simulink model "SAD_library"  (R2023b)
settings: Solver=VariableStepAuto  StartTime=0.0  StopTime=10.0  RelTol=1e-3
values from neighbouring files (symbols this model uses):
  A = 1e-2.*[6, 6, 6, 6, 4, 4, 12, 12, 12, 12]'    [SAD_project_code.m]
  e = 0.001    [SAD_project_code.m]
  FS = 800e-9    (= 8e-07)    [SAD_project_code.m]
  i = deg2rad(60)    [SAD_project_code.m]
  inc_tot = sqrt(inc_lin^2 + inc_acc^2)    [SAD_project_code.m]
  p = a*(1-e^2)    [SAD_project_code.m]
  R_E = astroConstants(23)    [SAD_project_code.m]
  ts_sensor = t_step    (= 0.01)    [SAD_project_code.m]
  w_E = deg2rad(15.04)/60/60    [SAD_project_code.m]
undefined symbols (not defined in the file or in its folder): A_1, A_10, A_2, A_3, A_4, A_5, A_6, A_7, A_8, A_9, gain_thdot, N_1, N_10, N_2, N_3, N_4, N_5, N_6, N_7, N_8, N_9, r_1, r_10, r_2, r_3, r_4, r_5, r_6, r_7, r_8, r_9, rho_d1, rho_d10, rho_d2, rho_d3, rho_d4, rho_d5, rho_d6, rho_d7, rho_d8, rho_d9, rho_s1, rho_s10, rho_s2, rho_s3, rho_s4, rho_s5, rho_s6, rho_s7, rho_s8, rho_s9
libraries: matrix_library x11
settings Model: Creator=samue  LastModifiedBy=rkomiii_masca

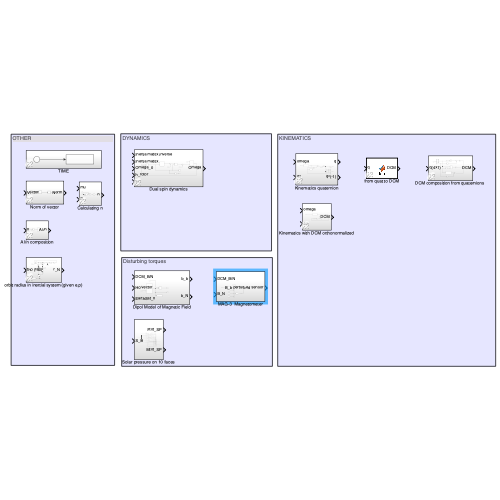
[thumbnail: Simulink's stored preview of the top-level diagram]
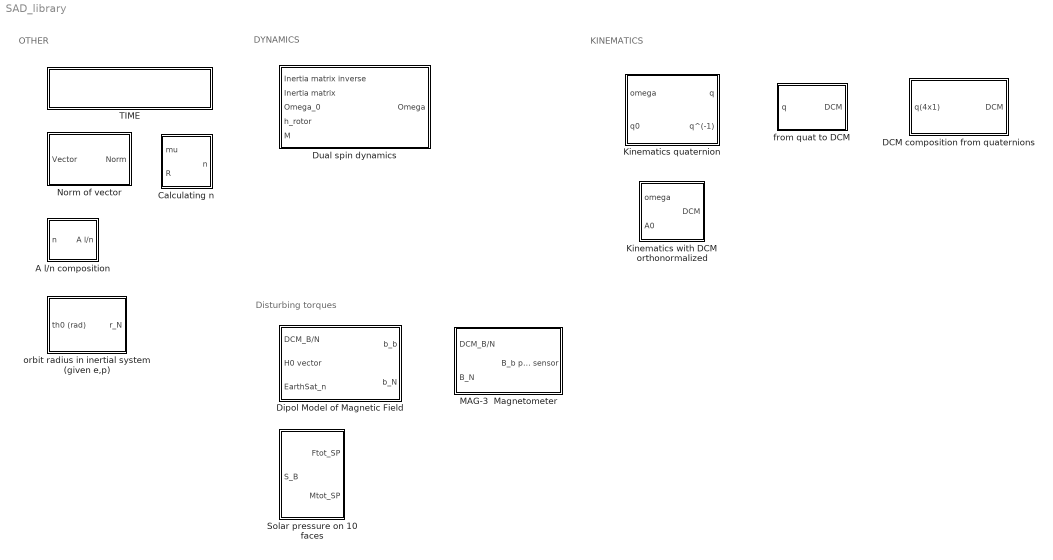
== system SAD_library ==
  note: KINEMATICS
  note: Disturbing torques
  note: OTHER
  note: DYNAMICS
  A l/n composition : Subsystem  AncestorBlock=LibrarySAD5/A l//n composition
  Calculating n : Subsystem  AncestorBlock=LibrarySAD5/Calculating n
  "DCM composition from quaternions " : Subsystem  AncestorBlock=LibrarySAD5/DCM composition from quaternions
  Dipol Model of Magnetic Field : Subsystem
  Dual spin dynamics : Subsystem  AncestorBlock=LibrarySAD5/Dual spin dynamics
  Kinematics quaternion : Subsystem  AncestorBlock=LibrarySAD5/Kinematics quaternion
  Kinematics with DCM orthonormalized : Subsystem  AncestorBlock=LibrarySAD5/Kinematics with DCM orthonormalized
  MAG-3  Magnetometer : Subsystem
  Norm of vector : Subsystem  AncestorBlock=LibrarySAD5/Normalize Vector1
  Solar pressure on 10 faces : Subsystem
  TIME : Subsystem  AncestorBlock=LibrarySAD5/TIME
  from quat to DCM : MATLAB Function  AncestorBlock=LibrarySAD5/from quat to DCM  TreatAsAtomicUnit=on
  orbit radius in inertial system (given e,p) : Subsystem  AncestorBlock=LibrarySAD5/orbit radius in inertial system (given e,p)

== system SAD_library/A l//n composition ==
  n : Inport
  Clock : Clock
  Product : Product
  Rotation matrix 3 : Subsystem
  A l/n : Outport
  wires:
  Rotation matrix 3/1(Out1) -> A l/n/1
  Product/1 -> Rotation matrix 3/1(In1)
  n/1 -> Product/1
  Clock/1 -> Product/2

== system SAD_library/Calculating n ==
  mu : Inport
  R : Inport  Port=2
  Divide : Product  Inputs=*/
  Product : Product  Inputs=3
  Sqrt : Sqrt
  n : Outport
  wires:
  Product/1 -> Divide/2
  Sqrt/1 -> n/1
  Divide/1 -> Sqrt/1
  mu/1 -> Divide/1
  R/1 -> Product/3, Product/2, Product/1

== system SAD_library/DCM composition from quaternions  ==
  q(4x1) : Inport
  Cross product matrix composition : Subsystem
  Demux : Demux
  Dot Product : DotProduct  OutDataTypeStr=Inherit: Inherit via internal rule
  Gain : Gain  Gain=[1 0 0; 0 1 0; 0 0 1]
  Gain1 : Gain  Gain=2
  Gain2 : Gain  Gain=-2
  Mux : Mux  Inputs=3
  Product : Product  Multiplication=Matrix(*)
  Product1 : Product
  Square : Math  Operator=square
  Sum : Sum  Inputs=|-+
  Sum1 : Sum  Inputs=+++
  Transpose : Math  Operator=transpose
  DCM : Outport
  wires:
  Gain/1 -> Sum1/1
  Demux/1 -> Mux/1
  q(4x1)/1 -> Demux/1
  Demux/2 -> Mux/2
  Mux/1 -> Dot Product/2, Dot Product/1, Product/1, Cross product matrix composition/1(q_vect), Transpose/1  "q_vect"
  Demux/4 -> Gain2/1, Square/1  "q4"
  Demux/3 -> Mux/3
  Dot Product/1 -> Sum/1
  Sum/1 -> Gain/1
  Square/1 -> Sum/2
  Transpose/1 -> Product/2
  Product/1 -> Gain1/1
  Gain2/1 -> Product1/2
  Cross product matrix composition/1(q_vect cross) -> Product1/1  "omega_mat"
  Product1/1 -> Sum1/3
  Gain1/1 -> Sum1/2
  Sum1/1 -> DCM/1

== system SAD_library/Dipol Model of Magnetic Field ==
  note: CODE TO ADD
      | % Definition of Magnetic Field (Dipole model)
      |  j_b = [0.01 0.05 0.01]';
      | H0 = 1e-9.*[-29404.8 -1450.9 4652.5]';
  DCM_B/N : Inport
  H0 vector : Inport  Port=2
  EarthSat_n : Inport  Port=3
  Calculation of b_n : Subsystem
  Matrix Multiply : Product  Multiplication=Matrix(*)
  To Workspace : ToWorkspace  VariableName=bn  SampleTime=-1
  b_b : Outport
  b_N : Outport  Port=2
  wires:
  Matrix Multiply/1 -> b_b/1
  DCM_B/N/1 -> Matrix Multiply/1
  H0 vector/1 -> Calculation of b_n/1(H0 vector)
  EarthSat_n/1 -> Calculation of b_n/2(EarthSat_n)
  Calculation of b_n/1(b_N) -> To Workspace/1, b_N/1, Matrix Multiply/2

== system SAD_library/Dual spin dynamics ==
  Inertia matrix inverse : Inport
  Inertia matrix : Inport  Port=2
  Omega_0 : Inport  Port=3
  h_rotor : Inport  Port=4
  M : Inport  Port=5
  Cross Product1 : matrix_library/Cross Product
  Integrator1 : Integrator  InitialConditionSource=external
  Product2 : Product  Multiplication=Matrix(*)
  Product3 : Product  Multiplication=Matrix(*)
  Scope2 : Scope
  Sum : Sum  Inputs=|++
  Sum1 : Sum  Inputs=|++
  Transpose : Math  Operator=transpose
  Omega : Outport
  wires:
  M/1 -> Sum1/2
  Sum1/1 -> Product3/2
  Omega_0/1 -> Integrator1/2
  Product2/1 -> Sum/1  "h"
  Inertia matrix/1 -> Product2/1
  Product3/1 -> Integrator1/1  "d_om/dt"
  h_rotor/1 -> Sum/2
  Integrator1/1 -> Product2/2, Cross Product1/2, Scope2/1, Transpose/1  "omega"
  Cross Product1/1 -> Sum1/1
  Inertia matrix inverse/1 -> Product3/1
  Sum/1 -> Cross Product1/1
  Transpose/1 -> Omega/1

== system SAD_library/Kinematics quaternion ==
  omega : Inport
  q0 : Inport  Port=2
  Demux : Demux
  Divide : Product  Inputs=*/
  Gain1 : Gain  Gain=-1
  Gain2 : Gain  Gain=-1
  Gain3 : Gain  Gain=1/2
  Gain5 : Gain  Gain=-1
  Integrator : Integrator  InitialConditionSource=external
  Matrix Multiply : Product  Multiplication=Matrix(*)
  Matrix OMEGA : Subsystem
  Mux : Mux
  Norm of Vector : Subsystem
  Scope : Scope
  q : Outport
  q^(-1) : Outport  Port=2
  wires:
  Gain3/1 -> Matrix Multiply/1  "1/2*Omega"
  Matrix Multiply/1 -> Integrator/1  "dq/dt"
  omega/1 -> Matrix OMEGA/1(omega)
  Integrator/1 -> Scope/1, q/1, Norm of Vector/1(Vector), Divide/1, Demux/1  "q"
  Matrix OMEGA/1(Matrix Omega) -> Gain3/1  "Omega"
  q0/1 -> Integrator/2
  Demux/2 -> Gain1/1
  Demux/3 -> Gain2/1
  Gain1/1 -> Mux/2
  Gain2/1 -> Mux/3
  Demux/4 -> Mux/4
  Mux/1 -> q^(-1)/1
  Norm of Vector/1(Norm) -> Divide/2  "q_norm"
  Divide/1 -> Matrix Multiply/2  "normalized q"
  Demux/1 -> Gain5/1
  Gain5/1 -> Mux/1

== system SAD_library/Kinematics with DCM orthonormalized ==
  omega : Inport
  A0 : Inport  Port=2
  Cross product matrix composition : Subsystem
  Integrator3 : Integrator  InitialConditionSource=external
  Orthonormalization of DCM : Subsystem
  Product1 : Product  Multiplication=Matrix(*)
  DCM : Outport
  wires:
  Integrator3/1 -> Orthonormalization of DCM/1(DCM), DCM/1  "DCM"
  Cross product matrix composition/1(omega cross) -> Product1/1  "omega cross"
  omega/1 -> Cross product matrix composition/1(omega)
  Orthonormalization of DCM/1(orthDCM) -> Product1/2
  Product1/1 -> Integrator3/1
  A0/1 -> Integrator3/2

== system SAD_library/MAG-3  Magnetometer ==
  note: CODE TO ADD TO MAKE SENSOR WORK
      | % Time definition
      | t0 = 0;
      | tf = T; %Period of orbit
      | t_step = 0.01; %fixed step of simulation
      | ts_sensor = t_step; % Sample of sensor (can change but must to be a multiple of t_step)
      |
      | % MAG-3 sensor data and error
      | FS = 500e-9; %Full scale value
      | inc_lin = 0.15/100; % Accuracy error
      | inc_acc = 0.75/100; % Linear error
      | inc_tot = sqrt(inc_lin^2 + inc_acc^2); %Total error
  DCM_B/N : Inport
  B_N : Inport  Port=2
  Error gain of sensor MAG-3 : Gain  Gain=inc_tot*FS
  Rotation in body frame : Product  Multiplication=Matrix(*)
  Sample of sensor : ZeroOrderHold  SampleTime=ts_sensor
  Saturation to FS : Saturate  UpperLimit=FS  LowerLimit=-FS
  Sum : Sum  Inputs=|++
  Vector Concatenate : Concatenate  NumInputs=3
  White Noise : RandomNumber  DisableCoverage=on  Seed=1  SampleTime=ts_sensor
  White Noise1 : RandomNumber  DisableCoverage=on  Seed=2  SampleTime=ts_sensor
  White Noise2 : RandomNumber  DisableCoverage=on  Seed=3  SampleTime=ts_sensor
  B_b perturbed sensor : Outport
  wires:
  Vector Concatenate/1 -> Error gain of sensor MAG-3/1
  White Noise/1 -> Vector Concatenate/1
  Error gain of sensor MAG-3/1 -> Sum/2
  White Noise2/1 -> Vector Concatenate/3
  White Noise1/1 -> Vector Concatenate/2
  Sum/1 -> Saturation to FS/1
  B_N/1 -> Sample of sensor/1
  DCM_B/N/1 -> Rotation in body frame/1
  Saturation to FS/1 -> B_b perturbed sensor/1
  Sample of sensor/1 -> Rotation in body frame/2
  Rotation in body frame/1 -> Sum/1

== system SAD_library/Norm of vector ==
  Vector : Inport
  Dot Product : DotProduct  OutDataTypeStr=Inherit: Inherit via internal rule
  Sqrt : Sqrt
  Norm : Outport
  wires:
  Sqrt/1 -> Norm/1
  Vector/1 -> Dot Product/1, Dot Product/2
  Dot Product/1 -> Sqrt/1

== system SAD_library/Solar pressure on 10 faces ==
  S_B : Inport
  Sum of forces : Sum  Inputs=++++++++++
  Sum of moments : Sum  Inputs=++++++++++
  solar pressure force and torque 1 : Subsystem
  solar pressure force and torque 10 : Subsystem
  solar pressure force and torque 2 : Subsystem
  solar pressure force and torque 3 : Subsystem
  solar pressure force and torque 4 : Subsystem
  solar pressure force and torque 5 : Subsystem
  solar pressure force and torque 6 : Subsystem
  solar pressure force and torque 7 : Subsystem
  solar pressure force and torque 8 : Subsystem
  solar pressure force and torque 9 : Subsystem
  Ftot_SP : Outport
  Mtot_SP : Outport  Port=2
  wires:
  solar pressure force and torque 1/1(F_1) -> Sum of forces/5
  solar pressure force and torque 2/1(F_2) -> Sum of forces/6
  solar pressure force and torque 3/1(F_3) -> Sum of forces/7
  solar pressure force and torque 4/1(F_4) -> Sum of forces/8
  solar pressure force and torque 5/1(F_5) -> Sum of forces/9
  solar pressure force and torque 6/1(F_6) -> Sum of forces/10
  solar pressure force and torque 7/1(F_7) -> Sum of forces/1
  solar pressure force and torque 8/1(F_8) -> Sum of forces/2
  solar pressure force and torque 9/1(F_9) -> Sum of forces/3
  solar pressure force and torque 10/1(F_10) -> Sum of forces/4
  solar pressure force and torque 1/2(M_1) -> Sum of moments/5
  solar pressure force and torque 2/2(M_2) -> Sum of moments/6
  solar pressure force and torque 3/2(M_3) -> Sum of moments/7
  solar pressure force and torque 4/2(M_4) -> Sum of moments/8
  solar pressure force and torque 5/2(M_5) -> Sum of moments/9
  solar pressure force and torque 6/2(M_6) -> Sum of moments/10
  solar pressure force and torque 7/2(M_7) -> Sum of moments/1
  solar pressure force and torque 8/2(M_8) -> Sum of moments/2
  solar pressure force and torque 9/2(M_9) -> Sum of moments/3
  solar pressure force and torque 10/2(M_10) -> Sum of moments/4
  Sum of forces/1 -> Ftot_SP/1  "Ftot_SP"
  Sum of moments/1 -> Mtot_SP/1  "Mtot_SP"
  S_B/1 -> solar pressure force and torque 10/1(s_B), solar pressure force and torque 9/1(s_B), solar pressure force and torque 6/1(s_B), solar pressure force and torque 5/1(s_B), solar pressure force and torque 4/1(s_B), solar pressure force and torque 7/1(s_B), solar pressure force and torque 8/1(s_B), solar pressure force and torque 1/1(s_B), solar pressure force and torque 2/1(s_B), solar pressure force and torque 3/1(s_B)

== system SAD_library/TIME ==
  Clock : Clock
  To Workspace1 : ToWorkspace  VariableName=t  SampleTime=-1
  wires:
  Clock/1 -> To Workspace1/1

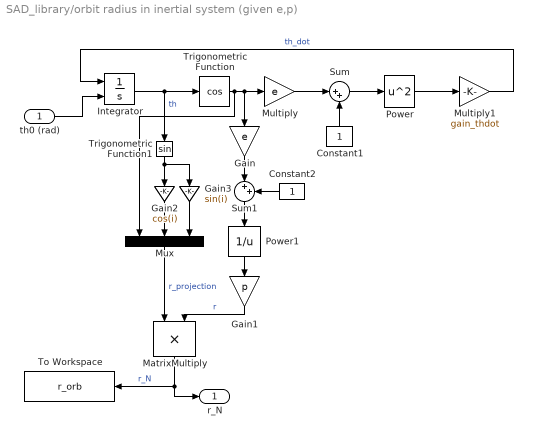
== system SAD_library/orbit radius in inertial system (given e,p) ==
  th0 (rad) : Inport
  Constant1 : Constant
  Constant2 : Constant
  Gain : Gain  Gain=e
  Gain1 : Gain  Gain=p
  Gain2 : Gain  Gain=cos(i)
  Gain3 : Gain  Gain=sin(i)
  Integrator : Integrator  InitialConditionSource=external
  MatrixMultiply : Product
  Multiply : Gain  Gain=e
  Multiply1 : Gain  Gain=gain_thdot
  Mux : Mux  Inputs=3
  Power : Math  Operator=square
  Power1 : Math  Operator=reciprocal
  Sum : Sum  Inputs=|++
  Sum1 : Sum  Inputs=|++
  To Workspace : ToWorkspace  VariableName=r_orb  SampleTime=-1
  Trigonometric Function : Trigonometry  Operator=cos
  Trigonometric Function1 : Trigonometry
  r_N : Outport
  wires:
  Mux/1 -> MatrixMultiply/1  "r_projection"
  Power1/1 -> Gain1/1
  Gain1/1 -> MatrixMultiply/2  "r"
  Gain2/1 -> Mux/2
  Sum1/1 -> Power1/1
  Constant2/1 -> Sum1/2
  Gain3/1 -> Mux/3
  th0 (rad)/1 -> Integrator/2
  Power/1 -> Multiply1/1
  MatrixMultiply/1 -> To Workspace/1, r_N/1  "r_N"
  Trigonometric Function1/1 -> Gain3/1, Gain2/1
  Multiply/1 -> Sum/1
  Gain/1 -> Sum1/1
  Multiply1/1 -> Integrator/1  "th_dot"
  Trigonometric Function/1 -> Mux/1, Gain/1, Multiply/1
  Sum/1 -> Power/1
  Integrator/1 -> Trigonometric Function1/1, Trigonometric Function/1  "th"
  Constant1/1 -> Sum/2

== system SAD_library/A l//n composition/Rotation matrix 3 ==
  In1 : Inport
  Constant1 : Constant  Value=[0 0 0; 0 0 0; 0 0 1]
  Cos2 : Trigonometry  Operator=cos
  Gain : Gain  Gain=[1 0 0; 0 1 0; 0 0 0]
  Gain1 : Gain  Gain=[0 1 0; -1 0 0; 0 0 0]
  Sin2 : Trigonometry
  Sum : Sum  Inputs=+++
  Out1 : Outport
  wires:
  Cos2/1 -> Gain/1
  Gain/1 -> Sum/1
  In1/1 -> Sin2/1, Cos2/1
  Sin2/1 -> Gain1/1
  Sum/1 -> Out1/1
  Gain1/1 -> Sum/2
  Constant1/1 -> Sum/3

== system SAD_library/DCM composition from quaternions /Cross product matrix composition ==
  q_vect : Inport
  Demux : Demux  Outputs=3
  Gain : Gain  Gain=[0 0 0; 0 0 -1; 0 1 0]
  Gain1 : Gain  Gain=[0 0 1; 0 0 0; -1 0 0]
  Gain2 : Gain  Gain=[0 -1 0; 1 0 0; 0 0 0]
  Sum : Sum  Inputs=+++
  q_vect cross : Outport
  wires:
  Gain1/1 -> Sum/2
  Demux/3 -> Gain2/1
  Demux/1 -> Gain/1
  q_vect/1 -> Demux/1
  Gain2/1 -> Sum/3
  Demux/2 -> Gain1/1
  Gain/1 -> Sum/1
  Sum/1 -> q_vect cross/1

== system SAD_library/Dipol Model of Magnetic Field/Calculation of b_n ==
  H0 vector : Inport
  EarthSat_n : Inport  Port=2
  Constant : Constant  Value=3
  Divide : Product  Inputs=*/
  Dot Product : DotProduct  OutDataTypeStr=Inherit: Inherit via internal rule
  Gain : Gain  Gain=3
  Gain1 : Gain  Gain=R_E^3
  Norm of vector : Subsystem  AncestorBlock=LibrarySAD5/Normalize Vector1
  Norm of vector1 : Subsystem  AncestorBlock=LibrarySAD5/Normalize Vector1
  Normalize Vector : Subsystem
  Power : Math  Operator=pow
  Product : Product
  Product1 : Product
  Subtract : Sum  Inputs=+-
  m_versor : Subsystem
  b_N : Outport
  wires:
  Norm of vector1/1(Norm) -> Power/1
  Product/1 -> Subtract/1
  Divide/1 -> Gain1/1
  EarthSat_n/1 -> Norm of vector1/1(Vector), Normalize Vector/1(Vector)
  Normalize Vector/1(Versor) -> Product/1, Dot Product/1
  Gain1/1 -> Product1/1
  m_versor/1(m_versor) -> Dot Product/2, Subtract/2
  Gain/1 -> Product/2
  Product1/1 -> b_N/1
  Constant/1 -> Power/2
  Dot Product/1 -> Gain/1
  Subtract/1 -> Product1/2
  Norm of vector/1(Norm) -> Divide/1
  Power/1 -> Divide/2
  H0 vector/1 -> Norm of vector/1(Vector)

== system SAD_library/Kinematics quaternion/Matrix OMEGA ==
  omega : Inport
  Demux1 : Demux  Outputs=3
  Gain3 : Gain  Gain=[0 0 0 1; 0 0 1 0; 0 -1 0 0; -1 0 0 0]
  Gain4 : Gain  Gain=[0 0 -1 0; 0 0 0 1; 1 0 0 0; 0 -1 0 0]
  Gain5 : Gain  Gain=[0 1 0 0; -1 0 0 0; 0 0 0 1; 0 0 -1 0]
  Sum : Sum  Inputs=+++
  Matrix Omega : Outport
  wires:
  Sum/1 -> Matrix Omega/1
  Demux1/3 -> Gain5/1
  Demux1/2 -> Gain4/1
  omega/1 -> Demux1/1
  Demux1/1 -> Gain3/1
  Gain3/1 -> Sum/1
  Gain4/1 -> Sum/2
  Gain5/1 -> Sum/3

== system SAD_library/Kinematics quaternion/Norm of Vector ==
  Vector : Inport
  Dot Product : DotProduct  OutDataTypeStr=Inherit: Inherit via internal rule
  Sqrt : Sqrt
  Norm : Outport
  wires:
  Sqrt/1 -> Norm/1
  Vector/1 -> Dot Product/1, Dot Product/2
  Dot Product/1 -> Sqrt/1

== system SAD_library/Kinematics with DCM orthonormalized/Cross product matrix composition ==
  omega : Inport
  Demux : Demux  Outputs=3
  Gain : Gain  Gain=[0 0 0; 0 0 -1; 0 1 0]
  Gain1 : Gain  Gain=[0 0 1; 0 0 0; -1 0 0]
  Gain2 : Gain  Gain=[0 -1 0; 1 0 0; 0 0 0]
  Sum : Sum  Inputs=+++
  omega cross : Outport
  wires:
  Sum/1 -> omega cross/1
  Gain1/1 -> Sum/2
  Demux/3 -> Gain2/1
  Demux/1 -> Gain/1
  omega/1 -> Demux/1
  Gain2/1 -> Sum/3
  Demux/2 -> Gain1/1
  Gain/1 -> Sum/1

== system SAD_library/Kinematics with DCM orthonormalized/Orthonormalization of DCM ==
  DCM : Inport
  Gain : Gain  Gain=3/2
  Gain1 : Gain  Gain=1/2
  Product : Product  Inputs=3  Multiplication=Matrix(*)
  Sum : Sum  Inputs=|+-
  Transpose : Math  Operator=transpose
  orthDCM : Outport
  wires:
  Sum/1 -> orthDCM/1
  Product/1 -> Gain1/1
  Transpose/1 -> Product/2
  Gain1/1 -> Sum/2
  DCM/1 -> Product/3, Transpose/1, Product/1, Gain/1
  Gain/1 -> Sum/1

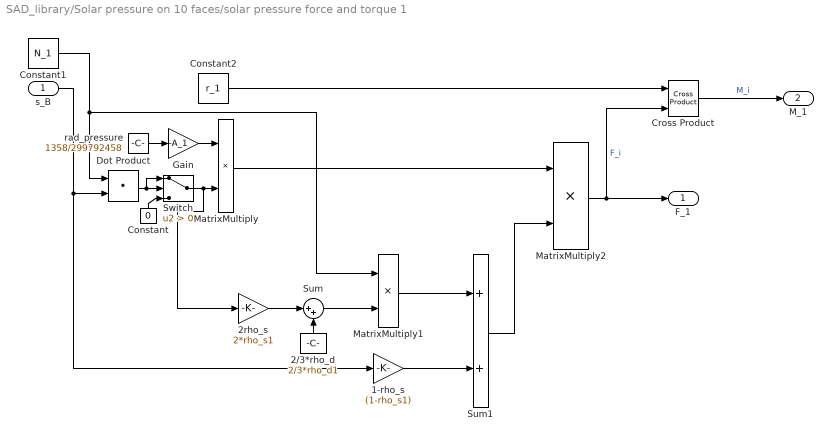
== system SAD_library/Solar pressure on 10 faces/solar pressure force and torque 1 ==
  s_B : Inport
  1-rho_s : Gain  Gain=(1-rho_s1)
  2/3*rho_d : Constant  Value=2/3*rho_d1
  2rho_s : Gain  Gain=2*rho_s1
  Constant : Constant  Value=0
  Constant1 : Constant  Value=N_1
  Constant2 : Constant  Value=r_1
  Cross Product : matrix_library/Cross Product
  Dot Product : DotProduct  OutDataTypeStr=Inherit: Inherit via internal rule
  Gain : Gain  Gain=-A_1
  MatrixMultiply : Product
  MatrixMultiply1 : Product
  MatrixMultiply2 : Product
  Sum : Sum  Inputs=|++
  Sum1 : Sum
  Switch : Switch  Criteria=u2 > Threshold  SaturateOnIntegerOverflow=off  InputSameDT=off
  rad_pressure : Constant  Value=1358/299792458
  F_1 : Outport
  M_1 : Outport  Port=2
  wires:
  MatrixMultiply2/1 -> Cross Product/2, F_1/1  "F_i"
  MatrixMultiply/1 -> MatrixMultiply2/1
  Sum1/1 -> MatrixMultiply2/2
  s_B/1 -> 1-rho_s/1, Dot Product/2
  2rho_s/1 -> Sum/1
  1-rho_s/1 -> Sum1/2
  rad_pressure/1 -> Gain/1
  2/3*rho_d/1 -> Sum/2
  MatrixMultiply1/1 -> Sum1/1
  Constant1/1 -> MatrixMultiply1/1, Dot Product/1
  Sum/1 -> MatrixMultiply1/2
  Gain/1 -> MatrixMultiply/1
  Constant2/1 -> Cross Product/1
  Cross Product/1 -> M_1/1  "M_i"
  Dot Product/1 -> Switch/1, Switch/2
  Constant/1 -> Switch/3
  Switch/1 -> 2rho_s/1, MatrixMultiply/2

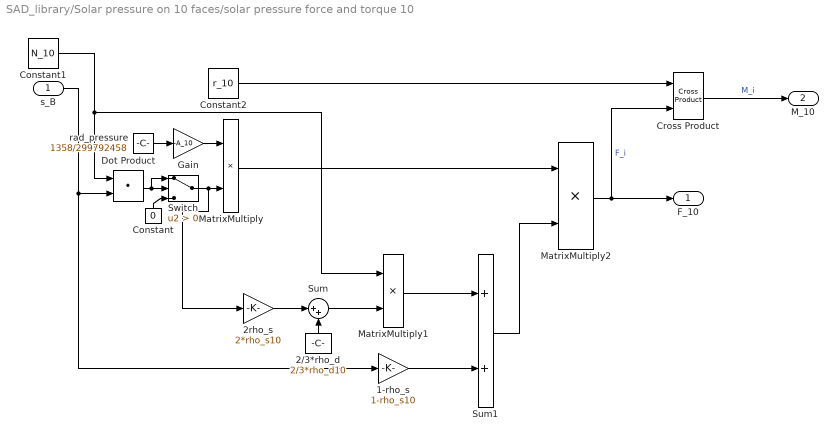
== system SAD_library/Solar pressure on 10 faces/solar pressure force and torque 10 ==
  s_B : Inport
  1-rho_s : Gain  Gain=1-rho_s10
  2/3*rho_d : Constant  Value=2/3*rho_d10
  2rho_s : Gain  Gain=2*rho_s10
  Constant : Constant  Value=0
  Constant1 : Constant  Value=N_10
  Constant2 : Constant  Value=r_10
  Cross Product : matrix_library/Cross Product
  Dot Product : DotProduct  OutDataTypeStr=Inherit: Inherit via internal rule
  Gain : Gain  Gain=-A_10
  MatrixMultiply : Product
  MatrixMultiply1 : Product
  MatrixMultiply2 : Product
  Sum : Sum  Inputs=|++
  Sum1 : Sum
  Switch : Switch  Criteria=u2 > Threshold  SaturateOnIntegerOverflow=off  InputSameDT=off
  rad_pressure : Constant  Value=1358/299792458
  F_10 : Outport
  M_10 : Outport  Port=2
  wires:
  MatrixMultiply2/1 -> Cross Product/2, F_10/1  "F_i"
  MatrixMultiply/1 -> MatrixMultiply2/1
  Sum1/1 -> MatrixMultiply2/2
  s_B/1 -> 1-rho_s/1, Dot Product/2
  2rho_s/1 -> Sum/1
  1-rho_s/1 -> Sum1/2
  rad_pressure/1 -> Gain/1
  2/3*rho_d/1 -> Sum/2
  MatrixMultiply1/1 -> Sum1/1
  Constant1/1 -> MatrixMultiply1/1, Dot Product/1
  Sum/1 -> MatrixMultiply1/2
  Gain/1 -> MatrixMultiply/1
  Constant2/1 -> Cross Product/1
  Cross Product/1 -> M_10/1  "M_i"
  Dot Product/1 -> Switch/1, Switch/2
  Constant/1 -> Switch/3
  Switch/1 -> 2rho_s/1, MatrixMultiply/2

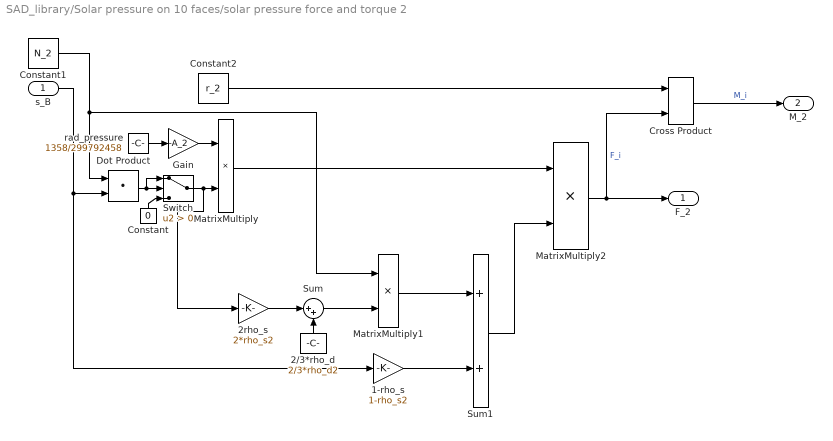
== system SAD_library/Solar pressure on 10 faces/solar pressure force and torque 2 ==
  s_B : Inport
  1-rho_s : Gain  Gain=1-rho_s2
  2/3*rho_d : Constant  Value=2/3*rho_d2
  2rho_s : Gain  Gain=2*rho_s2
  Constant : Constant  Value=0
  Constant1 : Constant  Value=N_2
  Constant2 : Constant  Value=r_2
  Cross Product : matrix_library/Cross Product
  Dot Product : DotProduct  OutDataTypeStr=Inherit: Inherit via internal rule
  Gain : Gain  Gain=-A_2
  MatrixMultiply : Product
  MatrixMultiply1 : Product
  MatrixMultiply2 : Product
  Sum : Sum  Inputs=|++
  Sum1 : Sum
  Switch : Switch  Criteria=u2 > Threshold  SaturateOnIntegerOverflow=off  InputSameDT=off
  rad_pressure : Constant  Value=1358/299792458
  F_2 : Outport
  M_2 : Outport  Port=2
  wires:
  MatrixMultiply2/1 -> Cross Product/2, F_2/1  "F_i"
  MatrixMultiply/1 -> MatrixMultiply2/1
  Sum1/1 -> MatrixMultiply2/2
  s_B/1 -> 1-rho_s/1, Dot Product/2
  2rho_s/1 -> Sum/1
  1-rho_s/1 -> Sum1/2
  rad_pressure/1 -> Gain/1
  2/3*rho_d/1 -> Sum/2
  MatrixMultiply1/1 -> Sum1/1
  Constant1/1 -> MatrixMultiply1/1, Dot Product/1
  Sum/1 -> MatrixMultiply1/2
  Gain/1 -> MatrixMultiply/1
  Constant2/1 -> Cross Product/1
  Cross Product/1 -> M_2/1  "M_i"
  Dot Product/1 -> Switch/1, Switch/2
  Constant/1 -> Switch/3
  Switch/1 -> 2rho_s/1, MatrixMultiply/2

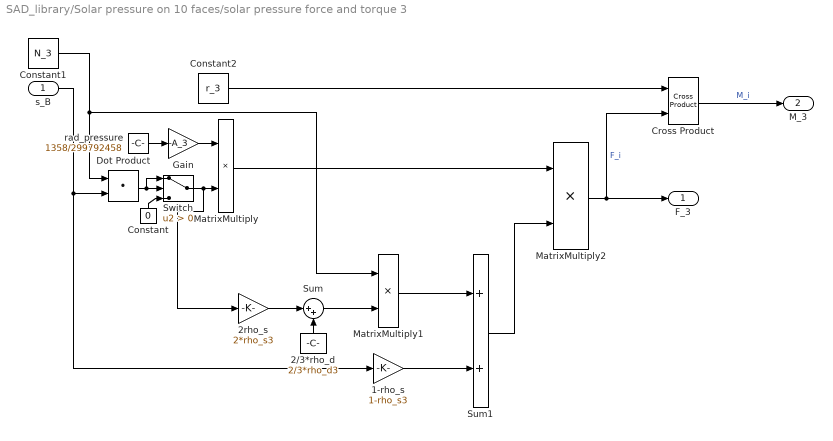
== system SAD_library/Solar pressure on 10 faces/solar pressure force and torque 3 ==
  s_B : Inport
  1-rho_s : Gain  Gain=1-rho_s3
  2/3*rho_d : Constant  Value=2/3*rho_d3
  2rho_s : Gain  Gain=2*rho_s3
  Constant : Constant  Value=0
  Constant1 : Constant  Value=N_3
  Constant2 : Constant  Value=r_3
  Cross Product : matrix_library/Cross Product
  Dot Product : DotProduct  OutDataTypeStr=Inherit: Inherit via internal rule
  Gain : Gain  Gain=-A_3
  MatrixMultiply : Product
  MatrixMultiply1 : Product
  MatrixMultiply2 : Product
  Sum : Sum  Inputs=|++
  Sum1 : Sum
  Switch : Switch  Criteria=u2 > Threshold  SaturateOnIntegerOverflow=off  InputSameDT=off
  rad_pressure : Constant  Value=1358/299792458
  F_3 : Outport
  M_3 : Outport  Port=2
  wires:
  MatrixMultiply2/1 -> Cross Product/2, F_3/1  "F_i"
  MatrixMultiply/1 -> MatrixMultiply2/1
  Sum1/1 -> MatrixMultiply2/2
  s_B/1 -> 1-rho_s/1, Dot Product/2
  2rho_s/1 -> Sum/1
  1-rho_s/1 -> Sum1/2
  rad_pressure/1 -> Gain/1
  2/3*rho_d/1 -> Sum/2
  MatrixMultiply1/1 -> Sum1/1
  Constant1/1 -> MatrixMultiply1/1, Dot Product/1
  Sum/1 -> MatrixMultiply1/2
  Gain/1 -> MatrixMultiply/1
  Constant2/1 -> Cross Product/1
  Cross Product/1 -> M_3/1  "M_i"
  Dot Product/1 -> Switch/1, Switch/2
  Constant/1 -> Switch/3
  Switch/1 -> 2rho_s/1, MatrixMultiply/2

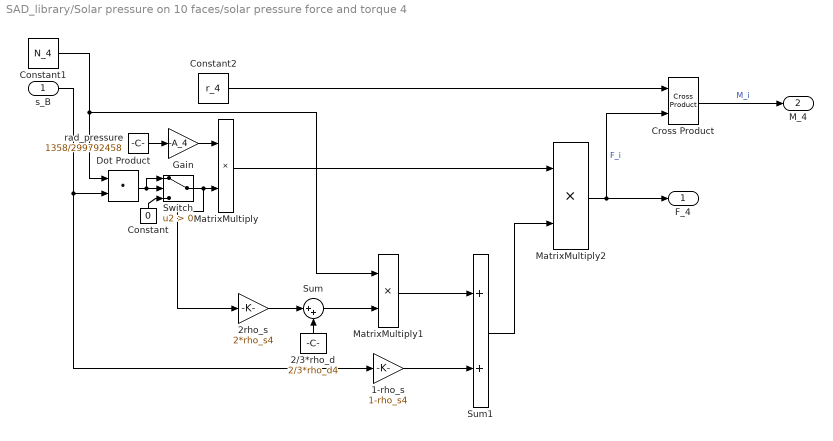
== system SAD_library/Solar pressure on 10 faces/solar pressure force and torque 4 ==
  s_B : Inport
  1-rho_s : Gain  Gain=1-rho_s4
  2/3*rho_d : Constant  Value=2/3*rho_d4
  2rho_s : Gain  Gain=2*rho_s4
  Constant : Constant  Value=0
  Constant1 : Constant  Value=N_4
  Constant2 : Constant  Value=r_4
  Cross Product : matrix_library/Cross Product
  Dot Product : DotProduct  OutDataTypeStr=Inherit: Inherit via internal rule
  Gain : Gain  Gain=-A_4
  MatrixMultiply : Product
  MatrixMultiply1 : Product
  MatrixMultiply2 : Product
  Sum : Sum  Inputs=|++
  Sum1 : Sum
  Switch : Switch  Criteria=u2 > Threshold  SaturateOnIntegerOverflow=off  InputSameDT=off
  rad_pressure : Constant  Value=1358/299792458
  F_4 : Outport
  M_4 : Outport  Port=2
  wires:
  MatrixMultiply2/1 -> Cross Product/2, F_4/1  "F_i"
  MatrixMultiply/1 -> MatrixMultiply2/1
  Sum1/1 -> MatrixMultiply2/2
  s_B/1 -> 1-rho_s/1, Dot Product/2
  2rho_s/1 -> Sum/1
  1-rho_s/1 -> Sum1/2
  rad_pressure/1 -> Gain/1
  2/3*rho_d/1 -> Sum/2
  MatrixMultiply1/1 -> Sum1/1
  Constant1/1 -> MatrixMultiply1/1, Dot Product/1
  Sum/1 -> MatrixMultiply1/2
  Gain/1 -> MatrixMultiply/1
  Constant2/1 -> Cross Product/1
  Cross Product/1 -> M_4/1  "M_i"
  Dot Product/1 -> Switch/1, Switch/2
  Constant/1 -> Switch/3
  Switch/1 -> 2rho_s/1, MatrixMultiply/2

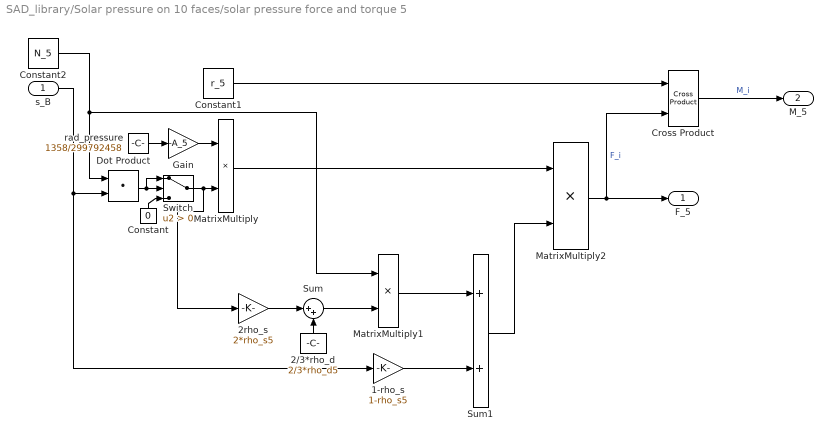
== system SAD_library/Solar pressure on 10 faces/solar pressure force and torque 5 ==
  s_B : Inport
  1-rho_s : Gain  Gain=1-rho_s5
  2/3*rho_d : Constant  Value=2/3*rho_d5
  2rho_s : Gain  Gain=2*rho_s5
  Constant : Constant  Value=0
  Constant1 : Constant  Value=r_5
  Constant2 : Constant  Value=N_5
  Cross Product : matrix_library/Cross Product
  Dot Product : DotProduct  OutDataTypeStr=Inherit: Inherit via internal rule
  Gain : Gain  Gain=-A_5
  MatrixMultiply : Product
  MatrixMultiply1 : Product
  MatrixMultiply2 : Product
  Sum : Sum  Inputs=|++
  Sum1 : Sum
  Switch : Switch  Criteria=u2 > Threshold  SaturateOnIntegerOverflow=off  InputSameDT=off
  rad_pressure : Constant  Value=1358/299792458
  F_5 : Outport
  M_5 : Outport  Port=2
  wires:
  MatrixMultiply2/1 -> Cross Product/2, F_5/1  "F_i"
  MatrixMultiply/1 -> MatrixMultiply2/1
  Sum1/1 -> MatrixMultiply2/2
  s_B/1 -> 1-rho_s/1, Dot Product/2
  2rho_s/1 -> Sum/1
  1-rho_s/1 -> Sum1/2
  rad_pressure/1 -> Gain/1
  2/3*rho_d/1 -> Sum/2
  MatrixMultiply1/1 -> Sum1/1
  Constant2/1 -> MatrixMultiply1/1, Dot Product/1
  Sum/1 -> MatrixMultiply1/2
  Gain/1 -> MatrixMultiply/1
  Constant1/1 -> Cross Product/1
  Cross Product/1 -> M_5/1  "M_i"
  Dot Product/1 -> Switch/1, Switch/2
  Constant/1 -> Switch/3
  Switch/1 -> 2rho_s/1, MatrixMultiply/2

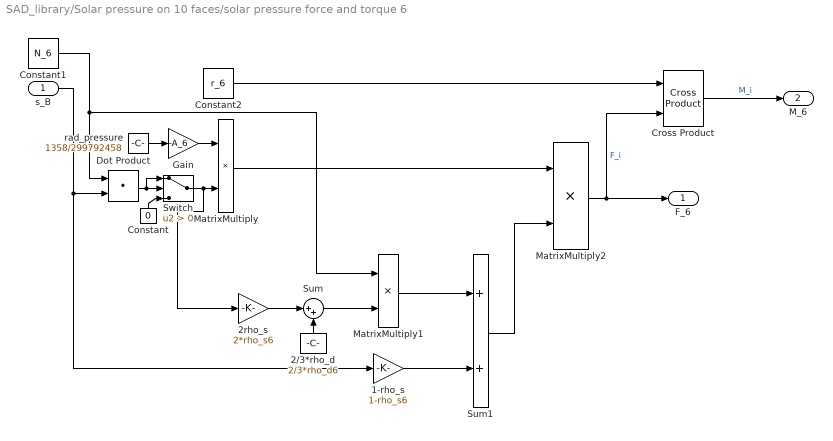
== system SAD_library/Solar pressure on 10 faces/solar pressure force and torque 6 ==
  s_B : Inport
  1-rho_s : Gain  Gain=1-rho_s6
  2/3*rho_d : Constant  Value=2/3*rho_d6
  2rho_s : Gain  Gain=2*rho_s6
  Constant : Constant  Value=0
  Constant1 : Constant  Value=N_6
  Constant2 : Constant  Value=r_6
  Cross Product : matrix_library/Cross Product
  Dot Product : DotProduct  OutDataTypeStr=Inherit: Inherit via internal rule
  Gain : Gain  Gain=-A_6
  MatrixMultiply : Product
  MatrixMultiply1 : Product
  MatrixMultiply2 : Product
  Sum : Sum  Inputs=|++
  Sum1 : Sum
  Switch : Switch  Criteria=u2 > Threshold  SaturateOnIntegerOverflow=off  InputSameDT=off
  rad_pressure : Constant  Value=1358/299792458
  F_6 : Outport
  M_6 : Outport  Port=2
  wires:
  MatrixMultiply2/1 -> Cross Product/2, F_6/1  "F_i"
  MatrixMultiply/1 -> MatrixMultiply2/1
  Sum1/1 -> MatrixMultiply2/2
  s_B/1 -> 1-rho_s/1, Dot Product/2
  2rho_s/1 -> Sum/1
  1-rho_s/1 -> Sum1/2
  rad_pressure/1 -> Gain/1
  2/3*rho_d/1 -> Sum/2
  MatrixMultiply1/1 -> Sum1/1
  Constant1/1 -> MatrixMultiply1/1, Dot Product/1
  Sum/1 -> MatrixMultiply1/2
  Gain/1 -> MatrixMultiply/1
  Constant2/1 -> Cross Product/1
  Cross Product/1 -> M_6/1  "M_i"
  Dot Product/1 -> Switch/1, Switch/2
  Constant/1 -> Switch/3
  Switch/1 -> 2rho_s/1, MatrixMultiply/2

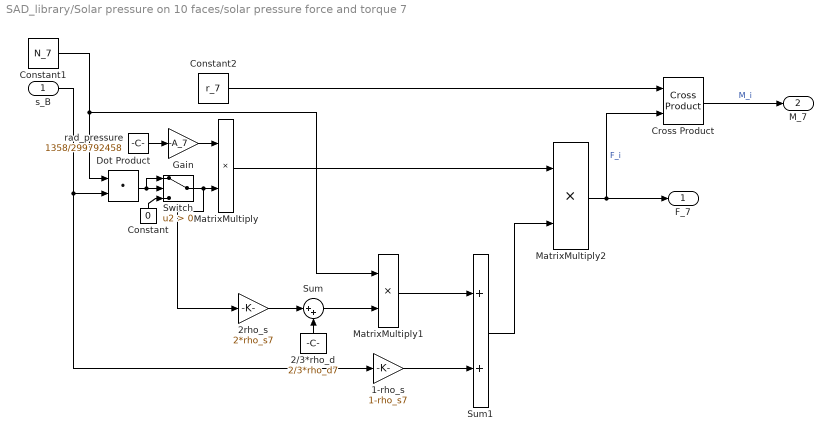
== system SAD_library/Solar pressure on 10 faces/solar pressure force and torque 7 ==
  s_B : Inport
  1-rho_s : Gain  Gain=1-rho_s7
  2/3*rho_d : Constant  Value=2/3*rho_d7
  2rho_s : Gain  Gain=2*rho_s7
  Constant : Constant  Value=0
  Constant1 : Constant  Value=N_7
  Constant2 : Constant  Value=r_7
  Cross Product : matrix_library/Cross Product
  Dot Product : DotProduct  OutDataTypeStr=Inherit: Inherit via internal rule
  Gain : Gain  Gain=-A_7
  MatrixMultiply : Product
  MatrixMultiply1 : Product
  MatrixMultiply2 : Product
  Sum : Sum  Inputs=|++
  Sum1 : Sum
  Switch : Switch  Criteria=u2 > Threshold  SaturateOnIntegerOverflow=off  InputSameDT=off
  rad_pressure : Constant  Value=1358/299792458
  F_7 : Outport
  M_7 : Outport  Port=2
  wires:
  MatrixMultiply2/1 -> Cross Product/2, F_7/1  "F_i"
  MatrixMultiply/1 -> MatrixMultiply2/1
  Sum1/1 -> MatrixMultiply2/2
  s_B/1 -> 1-rho_s/1, Dot Product/2
  2rho_s/1 -> Sum/1
  1-rho_s/1 -> Sum1/2
  rad_pressure/1 -> Gain/1
  2/3*rho_d/1 -> Sum/2
  MatrixMultiply1/1 -> Sum1/1
  Constant1/1 -> MatrixMultiply1/1, Dot Product/1
  Sum/1 -> MatrixMultiply1/2
  Gain/1 -> MatrixMultiply/1
  Constant2/1 -> Cross Product/1
  Cross Product/1 -> M_7/1  "M_i"
  Dot Product/1 -> Switch/1, Switch/2
  Constant/1 -> Switch/3
  Switch/1 -> 2rho_s/1, MatrixMultiply/2

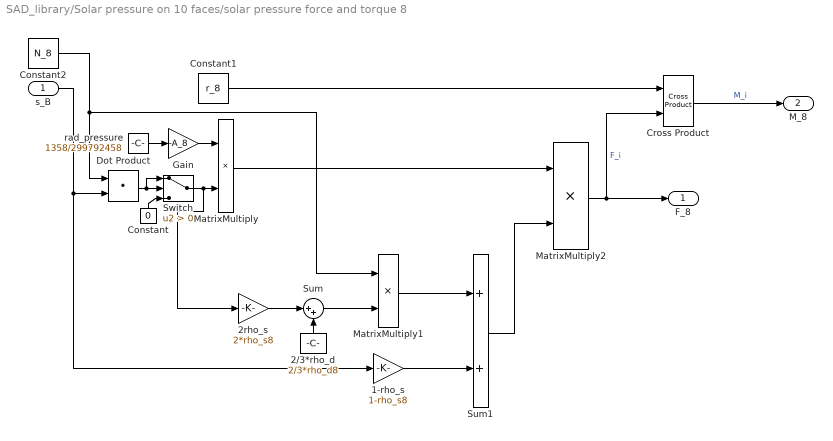
== system SAD_library/Solar pressure on 10 faces/solar pressure force and torque 8 ==
  s_B : Inport
  1-rho_s : Gain  Gain=1-rho_s8
  2/3*rho_d : Constant  Value=2/3*rho_d8
  2rho_s : Gain  Gain=2*rho_s8
  Constant : Constant  Value=0
  Constant1 : Constant  Value=r_8
  Constant2 : Constant  Value=N_8
  Cross Product : matrix_library/Cross Product
  Dot Product : DotProduct  OutDataTypeStr=Inherit: Inherit via internal rule
  Gain : Gain  Gain=-A_8
  MatrixMultiply : Product
  MatrixMultiply1 : Product
  MatrixMultiply2 : Product
  Sum : Sum  Inputs=|++
  Sum1 : Sum
  Switch : Switch  Criteria=u2 > Threshold  SaturateOnIntegerOverflow=off  InputSameDT=off
  rad_pressure : Constant  Value=1358/299792458
  F_8 : Outport
  M_8 : Outport  Port=2
  wires:
  MatrixMultiply2/1 -> Cross Product/2, F_8/1  "F_i"
  MatrixMultiply/1 -> MatrixMultiply2/1
  Sum1/1 -> MatrixMultiply2/2
  s_B/1 -> 1-rho_s/1, Dot Product/2
  2rho_s/1 -> Sum/1
  1-rho_s/1 -> Sum1/2
  rad_pressure/1 -> Gain/1
  2/3*rho_d/1 -> Sum/2
  MatrixMultiply1/1 -> Sum1/1
  Constant2/1 -> MatrixMultiply1/1, Dot Product/1
  Sum/1 -> MatrixMultiply1/2
  Gain/1 -> MatrixMultiply/1
  Constant1/1 -> Cross Product/1
  Cross Product/1 -> M_8/1  "M_i"
  Dot Product/1 -> Switch/1, Switch/2
  Constant/1 -> Switch/3
  Switch/1 -> 2rho_s/1, MatrixMultiply/2

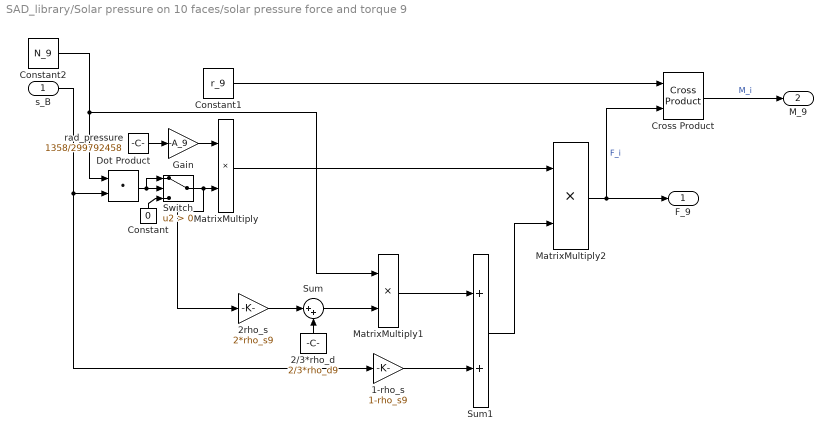
== system SAD_library/Solar pressure on 10 faces/solar pressure force and torque 9 ==
  s_B : Inport
  1-rho_s : Gain  Gain=1-rho_s9
  2/3*rho_d : Constant  Value=2/3*rho_d9
  2rho_s : Gain  Gain=2*rho_s9
  Constant : Constant  Value=0
  Constant1 : Constant  Value=r_9
  Constant2 : Constant  Value=N_9
  Cross Product : matrix_library/Cross Product
  Dot Product : DotProduct  OutDataTypeStr=Inherit: Inherit via internal rule
  Gain : Gain  Gain=-A_9
  MatrixMultiply : Product
  MatrixMultiply1 : Product
  MatrixMultiply2 : Product
  Sum : Sum  Inputs=|++
  Sum1 : Sum
  Switch : Switch  Criteria=u2 > Threshold  SaturateOnIntegerOverflow=off  InputSameDT=off
  rad_pressure : Constant  Value=1358/299792458
  F_9 : Outport
  M_9 : Outport  Port=2
  wires:
  MatrixMultiply2/1 -> Cross Product/2, F_9/1  "F_i"
  MatrixMultiply/1 -> MatrixMultiply2/1
  Sum1/1 -> MatrixMultiply2/2
  s_B/1 -> 1-rho_s/1, Dot Product/2
  2rho_s/1 -> Sum/1
  1-rho_s/1 -> Sum1/2
  rad_pressure/1 -> Gain/1
  2/3*rho_d/1 -> Sum/2
  MatrixMultiply1/1 -> Sum1/1
  Constant2/1 -> MatrixMultiply1/1, Dot Product/1
  Sum/1 -> MatrixMultiply1/2
  Gain/1 -> MatrixMultiply/1
  Constant1/1 -> Cross Product/1
  Cross Product/1 -> M_9/1  "M_i"
  Dot Product/1 -> Switch/1, Switch/2
  Constant/1 -> Switch/3
  Switch/1 -> 2rho_s/1, MatrixMultiply/2

== system SAD_library/Dipol Model of Magnetic Field/Calculation of b_n/Norm of vector ==
  Vector : Inport
  Dot Product : DotProduct  OutDataTypeStr=Inherit: Inherit via internal rule
  Sqrt : Sqrt
  Norm : Outport
  wires:
  Sqrt/1 -> Norm/1
  Vector/1 -> Dot Product/1, Dot Product/2
  Dot Product/1 -> Sqrt/1

== system SAD_library/Dipol Model of Magnetic Field/Calculation of b_n/Norm of vector1 ==
  Vector : Inport
  Dot Product : DotProduct  OutDataTypeStr=Inherit: Inherit via internal rule
  Sqrt : Sqrt
  Norm : Outport
  wires:
  Sqrt/1 -> Norm/1
  Vector/1 -> Dot Product/1, Dot Product/2
  Dot Product/1 -> Sqrt/1

== system SAD_library/Dipol Model of Magnetic Field/Calculation of b_n/Normalize Vector ==
  Vector : Inport
  Divide : Product  Inputs=*/
  Norm of vector : Subsystem  AncestorBlock=LibrarySAD5/Normalize Vector1
  Versor : Outport
  wires:
  Vector/1 -> Norm of vector/1(Vector), Divide/1
  Divide/1 -> Versor/1
  Norm of vector/1(Norm) -> Divide/2

== system SAD_library/Dipol Model of Magnetic Field/Calculation of b_n/m_versor ==
  Clock : Clock
  Constant : Constant  Value=cos(deg2rad(11.5))
  Cos : Trigonometry  Operator=cos
  Gain : Gain  Gain=deg2rad(w_E)
  Gain1 : Gain  Gain=sin(deg2rad(11.5))
  Gain2 : Gain  Gain=sin(deg2rad(11.5))
  Sin : Trigonometry
  Vector Concatenate : Concatenate  NumInputs=3
  m_versor : Outport
  wires:
  Clock/1 -> Gain/1
  Gain/1 -> Sin/1, Cos/1
  Gain2/1 -> Vector Concatenate/2
  Vector Concatenate/1 -> m_versor/1
  Cos/1 -> Gain1/1
  Constant/1 -> Vector Concatenate/3
  Sin/1 -> Gain2/1
  Gain1/1 -> Vector Concatenate/1

== system SAD_library/Dipol Model of Magnetic Field/Calculation of b_n/Normalize Vector/Norm of vector ==
  Vector : Inport
  Dot Product : DotProduct  OutDataTypeStr=Inherit: Inherit via internal rule
  Sqrt : Sqrt
  Norm : Outport
  wires:
  Sqrt/1 -> Norm/1
  Vector/1 -> Dot Product/1, Dot Product/2
  Dot Product/1 -> Sqrt/1

== matlab function SAD_library/from quat to DCM ==
  data: q input; DCM output
function DCM = fcn(q)
    
    DCM = (q(4)^2 - q(1:3)'*q(1:3))*eye(3,3) + 2*q(1:3)*q(1:3)' - 2*q(4)*[0 -q(3) q(2); q(3) 0 -q(1); -q(2) q(1) 0];
